simulink model "IEEE39_IBR_FrequencyControl_Primary"  (R2024a)
settings: Solver=VariableStepAuto  StartTime=0.0  StopTime=30  RelTol=1e-3
InitFcn:
  | IEEE39data_FrencyControl_primary;
values from neighbouring files (symbols this model uses):
  Fref = 60    [IEEE39data_FrencyControl_primary.m]
  IBR_data = [ ... (first row only)    [IEEE39data_FrencyControl_primary.m]
  line = [     1	2	0.0035	0.0411	0.6987	0	100	22 ... (first row only)    [IEEE39data_FrencyControl_primary.m]
  Sbase = 1e6    (= 1000000)    [IEEE39data_FrencyControl_primary.m]
  Vbase = 22e3    (= 22000)    [IEEE39data_FrencyControl_primary.m]
undefined symbols (not defined in the file or in its folder): t_start_disturbance
libraries: spsThreePhaseVIMeasurementLib x61, spsThreePhasePISectionLineLib x34, spsControlledVoltageSourceLib x33, spsabctodq0Lib x33, powerlib_extras x27, spsPLL3phLib x26, spsGroundLib x22, spsThreePhaseSeriesRLCBranchLib x22, spsThreePhaseParallelRLCLoadLib x20, slpidlib x14, spsMeanLib x11, spsdq0toabcLib x11
(part 4 of 5)

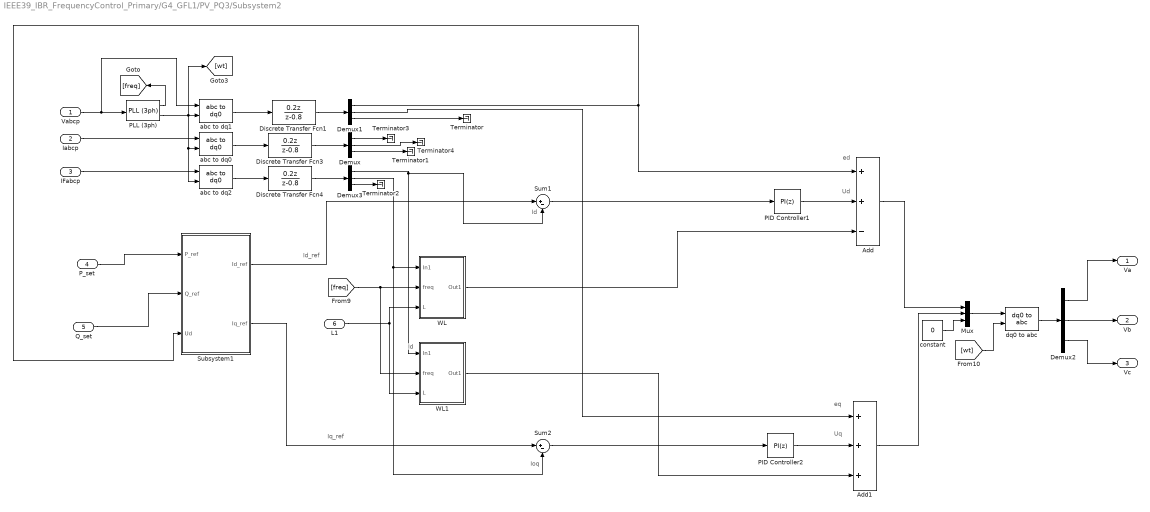
== system IEEE39_IBR_FrequencyControl_Primary/G4_GFL1/PV_PQ3/Subsystem2 ==
  note: Iq_ref
  note: Id
  note: Id_ref
  note: Ud
  note: Uq
  note: eq
  note: ed
  note: Ioq
  note: Id
  Vabcp : Inport
  Iabcp : Inport  Port=2
  IFabcp : Inport  Port=3
  P_set : Inport  Port=4
  Q_set : Inport  Port=5
  L1 : Inport  Port=6
  Add : Sum  Inputs=++-
  Add1 : Sum  Inputs=+++
  Demux{,1..3} (4 alike) : Demux  Outputs=3
  Discrete Transfer Fcn1 : DiscreteTransferFcn  Numerator=[0.2 0]  Denominator=[1 -0.8]  InitialStates=[1 1 1]  SampleTime=5e-4
  Discrete Transfer Fcn3 : DiscreteTransferFcn  Numerator=[0.2 0]  Denominator=[1 -0.8]  SampleTime=5e-4
  Discrete Transfer Fcn4 : DiscreteTransferFcn  Numerator=[0.2 0]  Denominator=[1 -0.8]  SampleTime=5e-4
  Mux : Mux  Inputs=3
  PID Controller1 : slpidlib/PID Controller  Controller=PI  Form=Parallel  TimeDomain=Discrete-time  UseExternalTs=off  SampleTime=5e-4  IntegratorMethod=Forward Euler  FilterMethod=Forward Euler  ControllerParametersSource=internal  P=50  I=400  UseKiTs=off  D=0  UseExternalDerivativeSource=off  N=100  UseFilter=on  TunerSelectOption=Transfer Function Based (PID Tuner App)  InitialConditionSource=internal  InitialConditionForIntegrator=0  InitialConditionForFilter=0  DifferentiatorICPrevScaledInput=0  ExternalReset=none  TrackingMode=off  Kt=1  LimitOutput=off  SatLimitsSource=internal  UpperSaturationLimit=inf  LowerSaturationLimit=-inf  LinearizeAsGain=on  AntiWindupMode=none  Kb=1  LimitIntegrator=off  UpperIntegratorSaturationLimit=inf  LowerIntegratorSaturationLimit=-inf  POutMin=[]  POutMax=[]  IOutMin=[]  IOutMax=[]  DOutMin=[]  DOutMax=[]  NOutMin=[]  NOutMax=[]  SumOutMin=[]  SumOutMax=[]  SaturationOutMin=[]  SaturationOutMax=[]  PParamMin=[]  PParamMax=[]  IParamMin=[]  IParamMax=[]  DParamMin=[]  DParamMax=[]  NParamMin=[]  NParamMax=[]  KbParamMin=[]  KbParamMax=[]  KtParamMin=[]  KtParamMax=[]  KbOutMin=[]  KbOutMax=[]  KtOutMin=[]  KtOutMax=[]  IntegratorOutMin=[]  IntegratorOutMax=[]  FilterOutMin=[]  FilterOutMax=[]  SumI1OutMin=[]  SumI1OutMax=[]  SumI2OutMin=[]  SumI2OutMax=[]  SumI3OutMin=[]  SumI3OutMax=[]  SumI4OutMin=[]  SumI4OutMax=[]  SumDOutMin=[]  SumDOutMax=[]  DifferentiatorOutMin=[]  DifferentiatorOutMax=[]  FilterDiffOutCoefMin=[]  FilterDiffOutCoefMax=[]  ReciprocalOutMin=[]  ReciprocalOutMax=[]  SumDenOutMin=[]  SumDenOutMax=[]  SumNumOutMin=[]  SumNumOutMax=[]  DivideOutMin=[]  DivideOutMax=[]  UdiffTsProdOutMin=[]  UdiffTsProdOutMax=[]  NTsProdOutMin=[]  NTsProdOutMax=[]  UintegralTsProdOutMin=[]  UintegralTsProdOutMax=[]  UngainTsProdOutMin=[]  UngainTsProdOutMax=[]  ClampingZeroOutDataTypeStr=Inherit: Inherit via back propagation  ClampingZeroOutMin=[]  ClampingZeroOutMax=[]  FilterDenConstantOutDataTypeStr=Inherit: Inherit via back propagation  FilterDenConstantOutMin=[]  FilterDenConstantOutMax=[]  PCopyOutDataTypeStr=Inherit: Inherit via back propagation  PCopyOutMin=[]  PCopyOutMax=[]  NCopyOutDataTypeStr=Inherit: Inherit via back propagation  NCopyOutMin=[]  NCopyOutMax=[]  IntegratorContinuousStateAttributes=''  IntegratorStateMustResolveToSignalObject=off  IntegratorRTWStateStorageClass=Auto  FilterContinuousStateAttributes=''  FilterStateMustResolveToSignalObject=off  FilterRTWStateStorageClass=Auto  ParallelPVariant=InternalParameters  IdealPVariant=Disabled  IVariant=InternalParameters  DVariant=Disabled  IntegratorVariant=Discrete  SatVariant=Disabled  AWVariant=Passthrough  PCopyVariant=Disabled  TRVariant=Disabled  FdbkBlocksVariant=Forward  IdealPFdbkVariant=Disabled  SatFdbkVariant=Disabled  DerivativeFilterVariant=Disabled  NVariant=Disabled  NCopyVariant=Disabled_SignalSpec  FilterICVariant=Disabled  IntegratorICVariant=InternalICs  ExternalResetVariant=Disabled  TRSumVariant=Passthrough  SumFdbkVariant=Disabled  SumVariant=Sum_PI  TsampFilterVariant=InternalTs  TsampNgainVariant=Passthrough  TsampIntegralVariant=Disabled_SignalSpec  ExternalSaturationOutDataTypeStr=Inherit: Same as second input  DerivativeSourceVariant=Disabled
  PID Controller2 : slpidlib/PID Controller  Controller=PI  Form=Parallel  TimeDomain=Discrete-time  UseExternalTs=off  SampleTime=5e-4  IntegratorMethod=Forward Euler  FilterMethod=Forward Euler  ControllerParametersSource=internal  P=50  I=400  UseKiTs=off  D=0  UseExternalDerivativeSource=off  N=100  UseFilter=on  TunerSelectOption=Transfer Function Based (PID Tuner App)  InitialConditionSource=internal  InitialConditionForIntegrator=0  InitialConditionForFilter=0  DifferentiatorICPrevScaledInput=0  ExternalReset=none  TrackingMode=off  Kt=1  LimitOutput=off  SatLimitsSource=internal  UpperSaturationLimit=inf  LowerSaturationLimit=-inf  LinearizeAsGain=on  AntiWindupMode=none  Kb=1  LimitIntegrator=off  UpperIntegratorSaturationLimit=inf  LowerIntegratorSaturationLimit=-inf  POutMin=[]  POutMax=[]  IOutMin=[]  IOutMax=[]  DOutMin=[]  DOutMax=[]  NOutMin=[]  NOutMax=[]  SumOutMin=[]  SumOutMax=[]  SaturationOutMin=[]  SaturationOutMax=[]  PParamMin=[]  PParamMax=[]  IParamMin=[]  IParamMax=[]  DParamMin=[]  DParamMax=[]  NParamMin=[]  NParamMax=[]  KbParamMin=[]  KbParamMax=[]  KtParamMin=[]  KtParamMax=[]  KbOutMin=[]  KbOutMax=[]  KtOutMin=[]  KtOutMax=[]  IntegratorOutMin=[]  IntegratorOutMax=[]  FilterOutMin=[]  FilterOutMax=[]  SumI1OutMin=[]  SumI1OutMax=[]  SumI2OutMin=[]  SumI2OutMax=[]  SumI3OutMin=[]  SumI3OutMax=[]  SumI4OutMin=[]  SumI4OutMax=[]  SumDOutMin=[]  SumDOutMax=[]  DifferentiatorOutMin=[]  DifferentiatorOutMax=[]  FilterDiffOutCoefMin=[]  FilterDiffOutCoefMax=[]  ReciprocalOutMin=[]  ReciprocalOutMax=[]  SumDenOutMin=[]  SumDenOutMax=[]  SumNumOutMin=[]  SumNumOutMax=[]  DivideOutMin=[]  DivideOutMax=[]  UdiffTsProdOutMin=[]  UdiffTsProdOutMax=[]  NTsProdOutMin=[]  NTsProdOutMax=[]  UintegralTsProdOutMin=[]  UintegralTsProdOutMax=[]  UngainTsProdOutMin=[]  UngainTsProdOutMax=[]  ClampingZeroOutDataTypeStr=Inherit: Inherit via back propagation  ClampingZeroOutMin=[]  ClampingZeroOutMax=[]  FilterDenConstantOutDataTypeStr=Inherit: Inherit via back propagation  FilterDenConstantOutMin=[]  FilterDenConstantOutMax=[]  PCopyOutDataTypeStr=Inherit: Inherit via back propagation  PCopyOutMin=[]  PCopyOutMax=[]  NCopyOutDataTypeStr=Inherit: Inherit via back propagation  NCopyOutMin=[]  NCopyOutMax=[]  IntegratorContinuousStateAttributes=''  IntegratorStateMustResolveToSignalObject=off  IntegratorRTWStateStorageClass=Auto  FilterContinuousStateAttributes=''  FilterStateMustResolveToSignalObject=off  FilterRTWStateStorageClass=Auto  ParallelPVariant=InternalParameters  IdealPVariant=Disabled  IVariant=InternalParameters  DVariant=Disabled  IntegratorVariant=Discrete  SatVariant=Disabled  AWVariant=Passthrough  PCopyVariant=Disabled  TRVariant=Disabled  FdbkBlocksVariant=Forward  IdealPFdbkVariant=Disabled  SatFdbkVariant=Disabled  DerivativeFilterVariant=Disabled  NVariant=Disabled  NCopyVariant=Disabled_SignalSpec  FilterICVariant=Disabled  IntegratorICVariant=InternalICs  ExternalResetVariant=Disabled  TRSumVariant=Passthrough  SumFdbkVariant=Disabled  SumVariant=Sum_PI  TsampFilterVariant=InternalTs  TsampNgainVariant=Passthrough  TsampIntegralVariant=Disabled_SignalSpec  ExternalSaturationOutDataTypeStr=Inherit: Same as second input  DerivativeSourceVariant=Disabled
  PLL (3ph) : spsPLL3phLib/PLL (3ph)  Fmin=59.5  Par_Init=[0, 60]  ParK=[180, 3200, 1]  TcD=1e-4  MaxRateChangeFreq=12  FilterCutOffFreq=25  Ts=1e-5  AGC=on
  Subsystem1 : Subsystem
  Sum1 : Sum  Inputs=|+-
  Sum2 : Sum  Inputs=|+-
  Terminator{,1..4} (5 alike) : Terminator
  WL : Subsystem
  WL1 : Subsystem
  abc to dq0 : spsabctodq0Lib/abc to dq0  Alignment=90 degrees behind phase A axis
  abc to dq1 : spsabctodq0Lib/abc to dq0  Alignment=90 degrees behind phase A axis
  abc to dq2 : spsabctodq0Lib/abc to dq0  Alignment=90 degrees behind phase A axis
  constant : Constant  Value=0
  dq0 to abc : spsdq0toabcLib/dq0 to abc  Alignment=90 degrees behind phase A axis
  Va : Outport  VectorParamsAs1DForOutWhenUnconnected=off
  Vb : Outport  Port=2  VectorParamsAs1DForOutWhenUnconnected=off
  Vc : Outport  Port=3  VectorParamsAs1DForOutWhenUnconnected=off
  wires:
  abc to dq0/1 -> Discrete Transfer Fcn3/1
  PLL (3ph)/2 -> [wt], abc to dq1/2, abc to dq2/2, abc to dq0/2
  Demux1/1 -> Add/1, Subsystem1/3(Ud)
  L1/1 -> WL/3(L), WL1/3(L)
  WL/1(Out1) -> Add/3
  [freq] -> WL1/2(freq), WL/2(freq)
  PLL (3ph)/1 -> [freq]
  Demux2/1 -> Va/1
  Add/1 -> Mux/1
  PID Controller2/1 -> Add1/2
  Demux2/2 -> Vb/1
  WL1/1(Out1) -> Add1/3
  Demux1/2 -> Add1/1
  Add1/1 -> Mux/2
  Mux/1 -> dq0 to abc/1
  Demux2/3 -> Vc/1
  dq0 to abc/1 -> Demux2/1
  Subsystem1/1(Id_ref) -> Sum1/1
  PID Controller1/1 -> Add/2
  [wt] -> dq0 to abc/2
  Subsystem1/2(Iq_ref) -> Sum2/1
  Demux1/3 -> Terminator/1
  Demux/3 -> Terminator1/1
  constant/1 -> Mux/3
  IFabcp/1 -> abc to dq2/1
  abc to dq2/1 -> Discrete Transfer Fcn4/1
  Demux3/3 -> Terminator2/1
  Demux3/2 -> Sum2/2, WL/1(In1)
  Demux3/1 -> Sum1/2, WL1/1(In1)
  Sum1/1 -> PID Controller1/1
  Sum2/1 -> PID Controller2/1
  P_set/1 -> Subsystem1/1(P_ref)
  Q_set/1 -> Subsystem1/2(Q_ref)
  Discrete Transfer Fcn3/1 -> Demux/1
  Discrete Transfer Fcn4/1 -> Demux3/1
  Demux/1 -> Terminator3/1
  Demux/2 -> Terminator4/1
  Discrete Transfer Fcn1/1 -> Demux1/1
  Iabcp/1 -> abc to dq0/1
  Vabcp/1 -> abc to dq1/1, PLL (3ph)/1
  abc to dq1/1 -> Discrete Transfer Fcn1/1

== system IEEE39_IBR_FrequencyControl_Primary/G5_GFL/PV_PQ3/Freq_Droop ==
  Pref : Inport
  Fref : Inport  Port=2
  Freq : Inport  Port=3
  D : Inport  Port=4
  Divide : Product  Inputs=*/
  Product : Product
  Product1 : Product
  S_base : Constant  Value=Sbase
  Saturation : Saturate  UpperLimit=10*Sbase  LowerLimit=0  ZeroCross=off
  Sum : Sum  Inputs=|+-
  Sum1 : Sum  Inputs=|+-
  Transfer Fcn : TransferFcn  Denominator=[0.318 1]
  Pset : Outport
  wires:
  Freq/1 -> Sum/1
  Fref/1 -> Sum/2, Divide/2
  S_base/1 -> Product/2
  D/1 -> Product1/1
  Product/1 -> Product1/2
  Pref/1 -> Sum1/1
  Product1/1 -> Sum1/2
  Saturation/1 -> Pset/1
  Sum1/1 -> Saturation/1
  Sum/1 -> Divide/1
  Transfer Fcn/1 -> Product/1
  Divide/1 -> Transfer Fcn/1

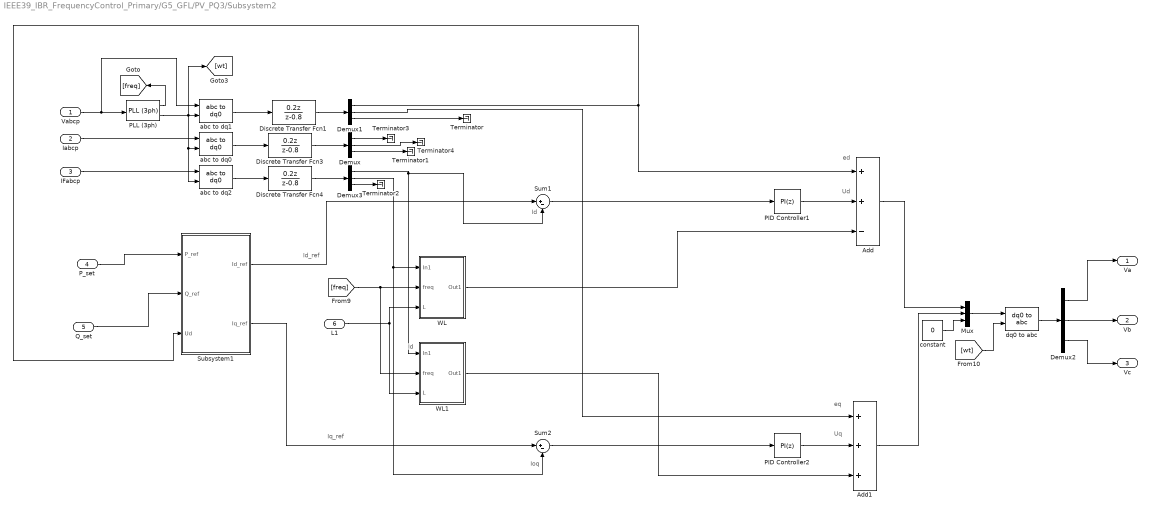
== system IEEE39_IBR_FrequencyControl_Primary/G5_GFL/PV_PQ3/Subsystem2 ==
  note: Iq_ref
  note: Id
  note: Id_ref
  note: Ud
  note: Uq
  note: eq
  note: ed
  note: Ioq
  note: Id
  Vabcp : Inport
  Iabcp : Inport  Port=2
  IFabcp : Inport  Port=3
  P_set : Inport  Port=4
  Q_set : Inport  Port=5
  L1 : Inport  Port=6
  Add : Sum  Inputs=++-
  Add1 : Sum  Inputs=+++
  Demux{,1..3} (4 alike) : Demux  Outputs=3
  Discrete Transfer Fcn1 : DiscreteTransferFcn  Numerator=[0.2 0]  Denominator=[1 -0.8]  InitialStates=[1 1 1]  SampleTime=5e-4
  Discrete Transfer Fcn3 : DiscreteTransferFcn  Numerator=[0.2 0]  Denominator=[1 -0.8]  SampleTime=5e-4
  Discrete Transfer Fcn4 : DiscreteTransferFcn  Numerator=[0.2 0]  Denominator=[1 -0.8]  SampleTime=5e-4
  Mux : Mux  Inputs=3
  PID Controller1 : slpidlib/PID Controller  Controller=PI  Form=Parallel  TimeDomain=Discrete-time  UseExternalTs=off  SampleTime=5e-4  IntegratorMethod=Forward Euler  FilterMethod=Forward Euler  ControllerParametersSource=internal  P=100  I=400  UseKiTs=off  D=0  UseExternalDerivativeSource=off  N=100  UseFilter=on  TunerSelectOption=Transfer Function Based (PID Tuner App)  InitialConditionSource=internal  InitialConditionForIntegrator=0  InitialConditionForFilter=0  DifferentiatorICPrevScaledInput=0  ExternalReset=none  TrackingMode=off  Kt=1  LimitOutput=off  SatLimitsSource=internal  UpperSaturationLimit=inf  LowerSaturationLimit=-inf  LinearizeAsGain=on  AntiWindupMode=none  Kb=1  LimitIntegrator=off  UpperIntegratorSaturationLimit=inf  LowerIntegratorSaturationLimit=-inf  POutMin=[]  POutMax=[]  IOutMin=[]  IOutMax=[]  DOutMin=[]  DOutMax=[]  NOutMin=[]  NOutMax=[]  SumOutMin=[]  SumOutMax=[]  SaturationOutMin=[]  SaturationOutMax=[]  PParamMin=[]  PParamMax=[]  IParamMin=[]  IParamMax=[]  DParamMin=[]  DParamMax=[]  NParamMin=[]  NParamMax=[]  KbParamMin=[]  KbParamMax=[]  KtParamMin=[]  KtParamMax=[]  KbOutMin=[]  KbOutMax=[]  KtOutMin=[]  KtOutMax=[]  IntegratorOutMin=[]  IntegratorOutMax=[]  FilterOutMin=[]  FilterOutMax=[]  SumI1OutMin=[]  SumI1OutMax=[]  SumI2OutMin=[]  SumI2OutMax=[]  SumI3OutMin=[]  SumI3OutMax=[]  SumI4OutMin=[]  SumI4OutMax=[]  SumDOutMin=[]  SumDOutMax=[]  DifferentiatorOutMin=[]  DifferentiatorOutMax=[]  FilterDiffOutCoefMin=[]  FilterDiffOutCoefMax=[]  ReciprocalOutMin=[]  ReciprocalOutMax=[]  SumDenOutMin=[]  SumDenOutMax=[]  SumNumOutMin=[]  SumNumOutMax=[]  DivideOutMin=[]  DivideOutMax=[]  UdiffTsProdOutMin=[]  UdiffTsProdOutMax=[]  NTsProdOutMin=[]  NTsProdOutMax=[]  UintegralTsProdOutMin=[]  UintegralTsProdOutMax=[]  UngainTsProdOutMin=[]  UngainTsProdOutMax=[]  ClampingZeroOutDataTypeStr=Inherit: Inherit via back propagation  ClampingZeroOutMin=[]  ClampingZeroOutMax=[]  FilterDenConstantOutDataTypeStr=Inherit: Inherit via back propagation  FilterDenConstantOutMin=[]  FilterDenConstantOutMax=[]  PCopyOutDataTypeStr=Inherit: Inherit via back propagation  PCopyOutMin=[]  PCopyOutMax=[]  NCopyOutDataTypeStr=Inherit: Inherit via back propagation  NCopyOutMin=[]  NCopyOutMax=[]  IntegratorContinuousStateAttributes=''  IntegratorStateMustResolveToSignalObject=off  IntegratorRTWStateStorageClass=Auto  FilterContinuousStateAttributes=''  FilterStateMustResolveToSignalObject=off  FilterRTWStateStorageClass=Auto  ParallelPVariant=InternalParameters  IdealPVariant=Disabled  IVariant=InternalParameters  DVariant=Disabled  IntegratorVariant=Discrete  SatVariant=Disabled  AWVariant=Passthrough  PCopyVariant=Disabled  TRVariant=Disabled  FdbkBlocksVariant=Forward  IdealPFdbkVariant=Disabled  SatFdbkVariant=Disabled  DerivativeFilterVariant=Disabled  NVariant=Disabled  NCopyVariant=Disabled_SignalSpec  FilterICVariant=Disabled  IntegratorICVariant=InternalICs  ExternalResetVariant=Disabled  TRSumVariant=Passthrough  SumFdbkVariant=Disabled  SumVariant=Sum_PI  TsampFilterVariant=InternalTs  TsampNgainVariant=Passthrough  TsampIntegralVariant=Disabled_SignalSpec  ExternalSaturationOutDataTypeStr=Inherit: Same as second input  DerivativeSourceVariant=Disabled
  PID Controller2 : slpidlib/PID Controller  Controller=PI  Form=Parallel  TimeDomain=Discrete-time  UseExternalTs=off  SampleTime=5e-4  IntegratorMethod=Forward Euler  FilterMethod=Forward Euler  ControllerParametersSource=internal  P=100  I=400  UseKiTs=off  D=0  UseExternalDerivativeSource=off  N=100  UseFilter=on  TunerSelectOption=Transfer Function Based (PID Tuner App)  InitialConditionSource=internal  InitialConditionForIntegrator=0  InitialConditionForFilter=0  DifferentiatorICPrevScaledInput=0  ExternalReset=none  TrackingMode=off  Kt=1  LimitOutput=off  SatLimitsSource=internal  UpperSaturationLimit=inf  LowerSaturationLimit=-inf  LinearizeAsGain=on  AntiWindupMode=none  Kb=1  LimitIntegrator=off  UpperIntegratorSaturationLimit=inf  LowerIntegratorSaturationLimit=-inf  POutMin=[]  POutMax=[]  IOutMin=[]  IOutMax=[]  DOutMin=[]  DOutMax=[]  NOutMin=[]  NOutMax=[]  SumOutMin=[]  SumOutMax=[]  SaturationOutMin=[]  SaturationOutMax=[]  PParamMin=[]  PParamMax=[]  IParamMin=[]  IParamMax=[]  DParamMin=[]  DParamMax=[]  NParamMin=[]  NParamMax=[]  KbParamMin=[]  KbParamMax=[]  KtParamMin=[]  KtParamMax=[]  KbOutMin=[]  KbOutMax=[]  KtOutMin=[]  KtOutMax=[]  IntegratorOutMin=[]  IntegratorOutMax=[]  FilterOutMin=[]  FilterOutMax=[]  SumI1OutMin=[]  SumI1OutMax=[]  SumI2OutMin=[]  SumI2OutMax=[]  SumI3OutMin=[]  SumI3OutMax=[]  SumI4OutMin=[]  SumI4OutMax=[]  SumDOutMin=[]  SumDOutMax=[]  DifferentiatorOutMin=[]  DifferentiatorOutMax=[]  FilterDiffOutCoefMin=[]  FilterDiffOutCoefMax=[]  ReciprocalOutMin=[]  ReciprocalOutMax=[]  SumDenOutMin=[]  SumDenOutMax=[]  SumNumOutMin=[]  SumNumOutMax=[]  DivideOutMin=[]  DivideOutMax=[]  UdiffTsProdOutMin=[]  UdiffTsProdOutMax=[]  NTsProdOutMin=[]  NTsProdOutMax=[]  UintegralTsProdOutMin=[]  UintegralTsProdOutMax=[]  UngainTsProdOutMin=[]  UngainTsProdOutMax=[]  ClampingZeroOutDataTypeStr=Inherit: Inherit via back propagation  ClampingZeroOutMin=[]  ClampingZeroOutMax=[]  FilterDenConstantOutDataTypeStr=Inherit: Inherit via back propagation  FilterDenConstantOutMin=[]  FilterDenConstantOutMax=[]  PCopyOutDataTypeStr=Inherit: Inherit via back propagation  PCopyOutMin=[]  PCopyOutMax=[]  NCopyOutDataTypeStr=Inherit: Inherit via back propagation  NCopyOutMin=[]  NCopyOutMax=[]  IntegratorContinuousStateAttributes=''  IntegratorStateMustResolveToSignalObject=off  IntegratorRTWStateStorageClass=Auto  FilterContinuousStateAttributes=''  FilterStateMustResolveToSignalObject=off  FilterRTWStateStorageClass=Auto  ParallelPVariant=InternalParameters  IdealPVariant=Disabled  IVariant=InternalParameters  DVariant=Disabled  IntegratorVariant=Discrete  SatVariant=Disabled  AWVariant=Passthrough  PCopyVariant=Disabled  TRVariant=Disabled  FdbkBlocksVariant=Forward  IdealPFdbkVariant=Disabled  SatFdbkVariant=Disabled  DerivativeFilterVariant=Disabled  NVariant=Disabled  NCopyVariant=Disabled_SignalSpec  FilterICVariant=Disabled  IntegratorICVariant=InternalICs  ExternalResetVariant=Disabled  TRSumVariant=Passthrough  SumFdbkVariant=Disabled  SumVariant=Sum_PI  TsampFilterVariant=InternalTs  TsampNgainVariant=Passthrough  TsampIntegralVariant=Disabled_SignalSpec  ExternalSaturationOutDataTypeStr=Inherit: Same as second input  DerivativeSourceVariant=Disabled
  PLL (3ph) : spsPLL3phLib/PLL (3ph)  Fmin=59.5  Par_Init=[0, 60]  ParK=[180, 3200, 1]  TcD=1e-4  MaxRateChangeFreq=12  FilterCutOffFreq=25  Ts=1e-5  AGC=on
  Subsystem1 : Subsystem
  Sum1 : Sum  Inputs=|+-
  Sum2 : Sum  Inputs=|+-
  Terminator{,1..4} (5 alike) : Terminator
  WL : Subsystem
  WL1 : Subsystem
  abc to dq0 : spsabctodq0Lib/abc to dq0  Alignment=90 degrees behind phase A axis
  abc to dq1 : spsabctodq0Lib/abc to dq0  Alignment=90 degrees behind phase A axis
  abc to dq2 : spsabctodq0Lib/abc to dq0  Alignment=90 degrees behind phase A axis
  constant : Constant  Value=0
  dq0 to abc : spsdq0toabcLib/dq0 to abc  Alignment=90 degrees behind phase A axis
  Va : Outport  VectorParamsAs1DForOutWhenUnconnected=off
  Vb : Outport  Port=2  VectorParamsAs1DForOutWhenUnconnected=off
  Vc : Outport  Port=3  VectorParamsAs1DForOutWhenUnconnected=off
  wires:
  abc to dq0/1 -> Discrete Transfer Fcn3/1
  PLL (3ph)/2 -> [wt], abc to dq1/2, abc to dq2/2, abc to dq0/2
  Demux1/1 -> Add/1, Subsystem1/3(Ud)
  L1/1 -> WL/3(L), WL1/3(L)
  WL/1(Out1) -> Add/3
  [freq] -> WL1/2(freq), WL/2(freq)
  PLL (3ph)/1 -> [freq]
  Demux2/1 -> Va/1
  Add/1 -> Mux/1
  PID Controller2/1 -> Add1/2
  Demux2/2 -> Vb/1
  WL1/1(Out1) -> Add1/3
  Demux1/2 -> Add1/1
  Add1/1 -> Mux/2
  Mux/1 -> dq0 to abc/1
  Demux2/3 -> Vc/1
  dq0 to abc/1 -> Demux2/1
  Subsystem1/1(Id_ref) -> Sum1/1
  PID Controller1/1 -> Add/2
  [wt] -> dq0 to abc/2
  Subsystem1/2(Iq_ref) -> Sum2/1
  Demux1/3 -> Terminator/1
  Demux/3 -> Terminator1/1
  constant/1 -> Mux/3
  IFabcp/1 -> abc to dq2/1
  abc to dq2/1 -> Discrete Transfer Fcn4/1
  Demux3/3 -> Terminator2/1
  Demux3/2 -> Sum2/2, WL/1(In1)
  Demux3/1 -> Sum1/2, WL1/1(In1)
  Sum1/1 -> PID Controller1/1
  Sum2/1 -> PID Controller2/1
  P_set/1 -> Subsystem1/1(P_ref)
  Q_set/1 -> Subsystem1/2(Q_ref)
  Discrete Transfer Fcn3/1 -> Demux/1
  Discrete Transfer Fcn4/1 -> Demux3/1
  Demux/1 -> Terminator3/1
  Demux/2 -> Terminator4/1
  Discrete Transfer Fcn1/1 -> Demux1/1
  Iabcp/1 -> abc to dq0/1
  Vabcp/1 -> abc to dq1/1, PLL (3ph)/1
  abc to dq1/1 -> Discrete Transfer Fcn1/1

== system IEEE39_IBR_FrequencyControl_Primary/G6_GFL/PV_PQ3/Freq_Droop ==
  Pref : Inport
  Fref : Inport  Port=2
  Freq : Inport  Port=3
  D : Inport  Port=4
  Divide : Product  Inputs=*/
  Product : Product
  Product1 : Product
  S_base : Constant  Value=Sbase
  Saturation : Saturate  UpperLimit=10*Sbase  LowerLimit=0  ZeroCross=off
  Sum : Sum  Inputs=|+-
  Sum1 : Sum  Inputs=|+-
  Transfer Fcn : TransferFcn  Denominator=[0.318 1]
  Pset : Outport
  wires:
  Freq/1 -> Sum/1
  Fref/1 -> Sum/2, Divide/2
  S_base/1 -> Product/2
  D/1 -> Product1/1
  Product/1 -> Product1/2
  Pref/1 -> Sum1/1
  Product1/1 -> Sum1/2
  Saturation/1 -> Pset/1
  Sum1/1 -> Saturation/1
  Sum/1 -> Divide/1
  Transfer Fcn/1 -> Product/1
  Divide/1 -> Transfer Fcn/1

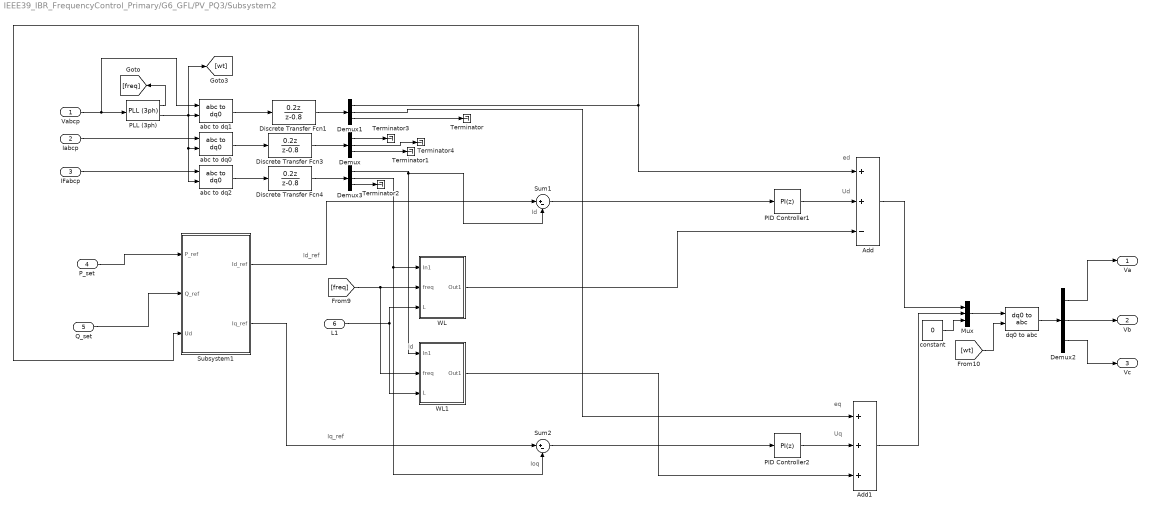
== system IEEE39_IBR_FrequencyControl_Primary/G6_GFL/PV_PQ3/Subsystem2 ==
  note: Iq_ref
  note: Id
  note: Id_ref
  note: Ud
  note: Uq
  note: eq
  note: ed
  note: Ioq
  note: Id
  Vabcp : Inport
  Iabcp : Inport  Port=2
  IFabcp : Inport  Port=3
  P_set : Inport  Port=4
  Q_set : Inport  Port=5
  L1 : Inport  Port=6
  Add : Sum  Inputs=++-
  Add1 : Sum  Inputs=+++
  Demux{,1..3} (4 alike) : Demux  Outputs=3
  Discrete Transfer Fcn1 : DiscreteTransferFcn  Numerator=[0.2 0]  Denominator=[1 -0.8]  InitialStates=[1 1 1]  SampleTime=5e-4
  Discrete Transfer Fcn3 : DiscreteTransferFcn  Numerator=[0.2 0]  Denominator=[1 -0.8]  SampleTime=5e-4
  Discrete Transfer Fcn4 : DiscreteTransferFcn  Numerator=[0.2 0]  Denominator=[1 -0.8]  SampleTime=5e-4
  Mux : Mux  Inputs=3
  PID Controller1 : slpidlib/PID Controller  Controller=PI  Form=Parallel  TimeDomain=Discrete-time  UseExternalTs=off  SampleTime=5e-4  IntegratorMethod=Forward Euler  FilterMethod=Forward Euler  ControllerParametersSource=internal  P=50  I=400  UseKiTs=off  D=0  UseExternalDerivativeSource=off  N=100  UseFilter=on  TunerSelectOption=Transfer Function Based (PID Tuner App)  InitialConditionSource=internal  InitialConditionForIntegrator=0  InitialConditionForFilter=0  DifferentiatorICPrevScaledInput=0  ExternalReset=none  TrackingMode=off  Kt=1  LimitOutput=off  SatLimitsSource=internal  UpperSaturationLimit=inf  LowerSaturationLimit=-inf  LinearizeAsGain=on  AntiWindupMode=none  Kb=1  LimitIntegrator=off  UpperIntegratorSaturationLimit=inf  LowerIntegratorSaturationLimit=-inf  POutMin=[]  POutMax=[]  IOutMin=[]  IOutMax=[]  DOutMin=[]  DOutMax=[]  NOutMin=[]  NOutMax=[]  SumOutMin=[]  SumOutMax=[]  SaturationOutMin=[]  SaturationOutMax=[]  PParamMin=[]  PParamMax=[]  IParamMin=[]  IParamMax=[]  DParamMin=[]  DParamMax=[]  NParamMin=[]  NParamMax=[]  KbParamMin=[]  KbParamMax=[]  KtParamMin=[]  KtParamMax=[]  KbOutMin=[]  KbOutMax=[]  KtOutMin=[]  KtOutMax=[]  IntegratorOutMin=[]  IntegratorOutMax=[]  FilterOutMin=[]  FilterOutMax=[]  SumI1OutMin=[]  SumI1OutMax=[]  SumI2OutMin=[]  SumI2OutMax=[]  SumI3OutMin=[]  SumI3OutMax=[]  SumI4OutMin=[]  SumI4OutMax=[]  SumDOutMin=[]  SumDOutMax=[]  DifferentiatorOutMin=[]  DifferentiatorOutMax=[]  FilterDiffOutCoefMin=[]  FilterDiffOutCoefMax=[]  ReciprocalOutMin=[]  ReciprocalOutMax=[]  SumDenOutMin=[]  SumDenOutMax=[]  SumNumOutMin=[]  SumNumOutMax=[]  DivideOutMin=[]  DivideOutMax=[]  UdiffTsProdOutMin=[]  UdiffTsProdOutMax=[]  NTsProdOutMin=[]  NTsProdOutMax=[]  UintegralTsProdOutMin=[]  UintegralTsProdOutMax=[]  UngainTsProdOutMin=[]  UngainTsProdOutMax=[]  ClampingZeroOutDataTypeStr=Inherit: Inherit via back propagation  ClampingZeroOutMin=[]  ClampingZeroOutMax=[]  FilterDenConstantOutDataTypeStr=Inherit: Inherit via back propagation  FilterDenConstantOutMin=[]  FilterDenConstantOutMax=[]  PCopyOutDataTypeStr=Inherit: Inherit via back propagation  PCopyOutMin=[]  PCopyOutMax=[]  NCopyOutDataTypeStr=Inherit: Inherit via back propagation  NCopyOutMin=[]  NCopyOutMax=[]  IntegratorContinuousStateAttributes=''  IntegratorStateMustResolveToSignalObject=off  IntegratorRTWStateStorageClass=Auto  FilterContinuousStateAttributes=''  FilterStateMustResolveToSignalObject=off  FilterRTWStateStorageClass=Auto  ParallelPVariant=InternalParameters  IdealPVariant=Disabled  IVariant=InternalParameters  DVariant=Disabled  IntegratorVariant=Discrete  SatVariant=Disabled  AWVariant=Passthrough  PCopyVariant=Disabled  TRVariant=Disabled  FdbkBlocksVariant=Forward  IdealPFdbkVariant=Disabled  SatFdbkVariant=Disabled  DerivativeFilterVariant=Disabled  NVariant=Disabled  NCopyVariant=Disabled_SignalSpec  FilterICVariant=Disabled  IntegratorICVariant=InternalICs  ExternalResetVariant=Disabled  TRSumVariant=Passthrough  SumFdbkVariant=Disabled  SumVariant=Sum_PI  TsampFilterVariant=InternalTs  TsampNgainVariant=Passthrough  TsampIntegralVariant=Disabled_SignalSpec  ExternalSaturationOutDataTypeStr=Inherit: Same as second input  DerivativeSourceVariant=Disabled
  PID Controller2 : slpidlib/PID Controller  Controller=PI  Form=Parallel  TimeDomain=Discrete-time  UseExternalTs=off  SampleTime=5e-4  IntegratorMethod=Forward Euler  FilterMethod=Forward Euler  ControllerParametersSource=internal  P=50  I=400  UseKiTs=off  D=0  UseExternalDerivativeSource=off  N=100  UseFilter=on  TunerSelectOption=Transfer Function Based (PID Tuner App)  InitialConditionSource=internal  InitialConditionForIntegrator=0  InitialConditionForFilter=0  DifferentiatorICPrevScaledInput=0  ExternalReset=none  TrackingMode=off  Kt=1  LimitOutput=off  SatLimitsSource=internal  UpperSaturationLimit=inf  LowerSaturationLimit=-inf  LinearizeAsGain=on  AntiWindupMode=none  Kb=1  LimitIntegrator=off  UpperIntegratorSaturationLimit=inf  LowerIntegratorSaturationLimit=-inf  POutMin=[]  POutMax=[]  IOutMin=[]  IOutMax=[]  DOutMin=[]  DOutMax=[]  NOutMin=[]  NOutMax=[]  SumOutMin=[]  SumOutMax=[]  SaturationOutMin=[]  SaturationOutMax=[]  PParamMin=[]  PParamMax=[]  IParamMin=[]  IParamMax=[]  DParamMin=[]  DParamMax=[]  NParamMin=[]  NParamMax=[]  KbParamMin=[]  KbParamMax=[]  KtParamMin=[]  KtParamMax=[]  KbOutMin=[]  KbOutMax=[]  KtOutMin=[]  KtOutMax=[]  IntegratorOutMin=[]  IntegratorOutMax=[]  FilterOutMin=[]  FilterOutMax=[]  SumI1OutMin=[]  SumI1OutMax=[]  SumI2OutMin=[]  SumI2OutMax=[]  SumI3OutMin=[]  SumI3OutMax=[]  SumI4OutMin=[]  SumI4OutMax=[]  SumDOutMin=[]  SumDOutMax=[]  DifferentiatorOutMin=[]  DifferentiatorOutMax=[]  FilterDiffOutCoefMin=[]  FilterDiffOutCoefMax=[]  ReciprocalOutMin=[]  ReciprocalOutMax=[]  SumDenOutMin=[]  SumDenOutMax=[]  SumNumOutMin=[]  SumNumOutMax=[]  DivideOutMin=[]  DivideOutMax=[]  UdiffTsProdOutMin=[]  UdiffTsProdOutMax=[]  NTsProdOutMin=[]  NTsProdOutMax=[]  UintegralTsProdOutMin=[]  UintegralTsProdOutMax=[]  UngainTsProdOutMin=[]  UngainTsProdOutMax=[]  ClampingZeroOutDataTypeStr=Inherit: Inherit via back propagation  ClampingZeroOutMin=[]  ClampingZeroOutMax=[]  FilterDenConstantOutDataTypeStr=Inherit: Inherit via back propagation  FilterDenConstantOutMin=[]  FilterDenConstantOutMax=[]  PCopyOutDataTypeStr=Inherit: Inherit via back propagation  PCopyOutMin=[]  PCopyOutMax=[]  NCopyOutDataTypeStr=Inherit: Inherit via back propagation  NCopyOutMin=[]  NCopyOutMax=[]  IntegratorContinuousStateAttributes=''  IntegratorStateMustResolveToSignalObject=off  IntegratorRTWStateStorageClass=Auto  FilterContinuousStateAttributes=''  FilterStateMustResolveToSignalObject=off  FilterRTWStateStorageClass=Auto  ParallelPVariant=InternalParameters  IdealPVariant=Disabled  IVariant=InternalParameters  DVariant=Disabled  IntegratorVariant=Discrete  SatVariant=Disabled  AWVariant=Passthrough  PCopyVariant=Disabled  TRVariant=Disabled  FdbkBlocksVariant=Forward  IdealPFdbkVariant=Disabled  SatFdbkVariant=Disabled  DerivativeFilterVariant=Disabled  NVariant=Disabled  NCopyVariant=Disabled_SignalSpec  FilterICVariant=Disabled  IntegratorICVariant=InternalICs  ExternalResetVariant=Disabled  TRSumVariant=Passthrough  SumFdbkVariant=Disabled  SumVariant=Sum_PI  TsampFilterVariant=InternalTs  TsampNgainVariant=Passthrough  TsampIntegralVariant=Disabled_SignalSpec  ExternalSaturationOutDataTypeStr=Inherit: Same as second input  DerivativeSourceVariant=Disabled
  PLL (3ph) : spsPLL3phLib/PLL (3ph)  Fmin=59.5  Par_Init=[0, 60]  ParK=[180, 3200, 1]  TcD=1e-4  MaxRateChangeFreq=12  FilterCutOffFreq=25  Ts=1e-5  AGC=on
  Subsystem1 : Subsystem
  Sum1 : Sum  Inputs=|+-
  Sum2 : Sum  Inputs=|+-
  Terminator{,1..4} (5 alike) : Terminator
  WL : Subsystem
  WL1 : Subsystem
  abc to dq0 : spsabctodq0Lib/abc to dq0  Alignment=90 degrees behind phase A axis
  abc to dq1 : spsabctodq0Lib/abc to dq0  Alignment=90 degrees behind phase A axis
  abc to dq2 : spsabctodq0Lib/abc to dq0  Alignment=90 degrees behind phase A axis
  constant : Constant  Value=0
  dq0 to abc : spsdq0toabcLib/dq0 to abc  Alignment=90 degrees behind phase A axis
  Va : Outport  VectorParamsAs1DForOutWhenUnconnected=off
  Vb : Outport  Port=2  VectorParamsAs1DForOutWhenUnconnected=off
  Vc : Outport  Port=3  VectorParamsAs1DForOutWhenUnconnected=off
  wires:
  abc to dq0/1 -> Discrete Transfer Fcn3/1
  PLL (3ph)/2 -> [wt], abc to dq1/2, abc to dq2/2, abc to dq0/2
  Demux1/1 -> Add/1, Subsystem1/3(Ud)
  L1/1 -> WL/3(L), WL1/3(L)
  WL/1(Out1) -> Add/3
  [freq] -> WL1/2(freq), WL/2(freq)
  PLL (3ph)/1 -> [freq]
  Demux2/1 -> Va/1
  Add/1 -> Mux/1
  PID Controller2/1 -> Add1/2
  Demux2/2 -> Vb/1
  WL1/1(Out1) -> Add1/3
  Demux1/2 -> Add1/1
  Add1/1 -> Mux/2
  Mux/1 -> dq0 to abc/1
  Demux2/3 -> Vc/1
  dq0 to abc/1 -> Demux2/1
  Subsystem1/1(Id_ref) -> Sum1/1
  PID Controller1/1 -> Add/2
  [wt] -> dq0 to abc/2
  Subsystem1/2(Iq_ref) -> Sum2/1
  Demux1/3 -> Terminator/1
  Demux/3 -> Terminator1/1
  constant/1 -> Mux/3
  IFabcp/1 -> abc to dq2/1
  abc to dq2/1 -> Discrete Transfer Fcn4/1
  Demux3/3 -> Terminator2/1
  Demux3/2 -> Sum2/2, WL/1(In1)
  Demux3/1 -> Sum1/2, WL1/1(In1)
  Sum1/1 -> PID Controller1/1
  Sum2/1 -> PID Controller2/1
  P_set/1 -> Subsystem1/1(P_ref)
  Q_set/1 -> Subsystem1/2(Q_ref)
  Discrete Transfer Fcn3/1 -> Demux/1
  Discrete Transfer Fcn4/1 -> Demux3/1
  Demux/1 -> Terminator3/1
  Demux/2 -> Terminator4/1
  Discrete Transfer Fcn1/1 -> Demux1/1
  Iabcp/1 -> abc to dq0/1
  Vabcp/1 -> abc to dq1/1, PLL (3ph)/1
  abc to dq1/1 -> Discrete Transfer Fcn1/1

== system IEEE39_IBR_FrequencyControl_Primary/GFM1/PV_PQ3/Freq_Droop ==
  Pref : Inport
  Fref : Inport  Port=2
  Pmeans : Inport  Port=3
  Add : Sum  Inputs=+-
  Add1 : Sum
  Divide : Product  Inputs=*/
  Product : Product
  S_base : Constant  Value=Sbase
  Saturation : Saturate  UpperLimit=2  LowerLimit=-2  ZeroCross=off
  Step : Step  Time=5  SampleTime=0
  Switch : Switch  Criteria=u2 > Threshold  SaturateOnIntegerOverflow=off  InputSameDT=off
  Transfer Fcn : TransferFcn  Denominator=[IBR_data(10,5) IBR_data(10,4)]
  Transfer Fcn1 : TransferFcn  Numerator=[20]  Denominator=[1 20]
  Transfer Fcn2 : TransferFcn  Denominator=[IBR_data(10,5) IBR_data(10,4)]
  fset : Outport
  wires:
  Pref/1 -> Add/1
  Transfer Fcn1/1 -> Add/2
  S_base/1 -> Divide/2
  Switch/1 -> Product/1
  Add1/1 -> fset/1
  Saturation/1 -> Add1/1
  Product/1 -> Saturation/1
  Add/1 -> Divide/1
  Pmeans/1 -> Transfer Fcn1/1
  Fref/1 -> Add1/2, Product/2
  Transfer Fcn2/1 -> Switch/1
  Transfer Fcn/1 -> Switch/3
  Step/1 -> Switch/2
  Divide/1 -> Transfer Fcn/1, Transfer Fcn2/1

== system IEEE39_IBR_FrequencyControl_Primary/GFM1/PV_PQ3/V//F ==
  vabcb : Inport
  iabcb : Inport  Port=2
  iFabcb : Inport  Port=3
  Vref_LL : Inport  Port=4
  f : Inport  Port=5
  Init_Phase_degree : Inport  Port=6
  Constant1 : Constant  Value=0
  Constant2 : Constant  Value=sqrt(2)/sqrt(3)
  Product : Product
  Subsystem : Subsystem
  UIcontrol : Subsystem
  Va : Outport
  Vb : Outport  Port=2
  Vc : Outport  Port=3
  wires:
  Constant1/1 -> UIcontrol/3(eq_ref)
  vabcb/1 -> Subsystem/1(eo)
  iFabcb/1 -> Subsystem/3(i)
  iabcb/1 -> Subsystem/2(io)
  Subsystem/1(eod) -> UIcontrol/2(ed)
  Subsystem/2(eoq) -> UIcontrol/4(eq)
  Subsystem/3(iod) -> UIcontrol/5(iod)
  Subsystem/4(ioq) -> UIcontrol/6(ioq)
  Subsystem/5(id) -> UIcontrol/7(id)
  Subsystem/6(iq) -> UIcontrol/8(iq)
  Subsystem/7(w) -> UIcontrol/9(w)
  UIcontrol/1(Va) -> Va/1
  UIcontrol/2(Vb) -> Vb/1
  UIcontrol/3(Vc) -> Vc/1
  f/1 -> Subsystem/4(f)
  Init_Phase_degree/1 -> Subsystem/5(Init_Phase_degree)
  Vref_LL/1 -> Product/1
  Product/1 -> UIcontrol/1(ed_ref)
  Constant2/1 -> Product/2
  Subsystem/8("wt ") -> UIcontrol/10("wt ")

== system IEEE39_IBR_FrequencyControl_Primary/GFM2/PV_PQ3/Freq_Droop ==
  Pref : Inport
  Fref : Inport  Port=2
  Pmeans : Inport  Port=3
  Add : Sum  Inputs=+-
  Add1 : Sum
  Divide : Product  Inputs=*/
  Product : Product
  S_base : Constant  Value=Sbase
  Saturation : Saturate  UpperLimit=2  LowerLimit=-2  ZeroCross=off
  Step : Step  Time=5  SampleTime=0
  Switch : Switch  Criteria=u2 > Threshold  SaturateOnIntegerOverflow=off  InputSameDT=off
  Transfer Fcn : TransferFcn  Denominator=[IBR_data(9,5) IBR_data(9,4)]
  Transfer Fcn1 : TransferFcn  Numerator=[20]  Denominator=[1 20]
  Transfer Fcn2 : TransferFcn  Denominator=[IBR_data(9,5) IBR_data(9,4)]
  fset : Outport
  wires:
  Pref/1 -> Add/1
  Transfer Fcn1/1 -> Add/2
  S_base/1 -> Divide/2
  Switch/1 -> Product/1
  Add1/1 -> fset/1
  Saturation/1 -> Add1/1
  Product/1 -> Saturation/1
  Add/1 -> Divide/1
  Pmeans/1 -> Transfer Fcn1/1
  Fref/1 -> Add1/2, Product/2
  Transfer Fcn2/1 -> Switch/1
  Transfer Fcn/1 -> Switch/3
  Step/1 -> Switch/2
  Divide/1 -> Transfer Fcn/1, Transfer Fcn2/1

== system IEEE39_IBR_FrequencyControl_Primary/GFM2/PV_PQ3/V//F ==
  vabcb : Inport
  iabcb : Inport  Port=2
  iFabcb : Inport  Port=3
  Vref_LL : Inport  Port=4
  f : Inport  Port=5
  Init_Phase_degree : Inport  Port=6
  Constant : Constant  Value=2*pi
  Constant1 : Constant  Value=0
  Constant2 : Constant  Value=sqrt(2)/sqrt(3)
  Divide : Product  Inputs=*/
  Product : Product
  Scope1 : Scope
  Subsystem : Subsystem
  UIcontrol : Subsystem
  Va : Outport
  Vb : Outport  Port=2
  Vc : Outport  Port=3
  wires:
  Constant1/1 -> UIcontrol/3(eq_ref)
  vabcb/1 -> Subsystem/1(eo)
  iFabcb/1 -> Subsystem/3(i)
  iabcb/1 -> Subsystem/2(io)
  Subsystem/1(eod) -> UIcontrol/2(ed)
  Subsystem/2(eoq) -> UIcontrol/4(eq)
  Subsystem/3(iod) -> UIcontrol/5(iod)
  Subsystem/4(ioq) -> UIcontrol/6(ioq)
  Subsystem/5(id) -> UIcontrol/7(id)
  Subsystem/6(iq) -> UIcontrol/8(iq)
  Subsystem/7(w) -> Divide/1, UIcontrol/9(w)
  UIcontrol/1(Va) -> Va/1
  UIcontrol/2(Vb) -> Vb/1
  UIcontrol/3(Vc) -> Vc/1
  f/1 -> Subsystem/4(f)
  Init_Phase_degree/1 -> Subsystem/5(Init_Phase_degree)
  Vref_LL/1 -> Product/1
  Product/1 -> UIcontrol/1(ed_ref)
  Constant2/1 -> Product/2
  Subsystem/8("wt ") -> UIcontrol/10("wt ")
  Constant/1 -> Divide/2
  Divide/1 -> Scope1/1

== system IEEE39_IBR_FrequencyControl_Primary/GFM3/PV_PQ3/Freq_Droop ==
  Pref : Inport
  Fref : Inport  Port=2
  Pmeans : Inport  Port=3
  Add : Sum  Inputs=+-
  Add1 : Sum
  Divide : Product  Inputs=*/
  Product : Product
  S_base : Constant  Value=Sbase
  Saturation : Saturate  UpperLimit=2  LowerLimit=-2  ZeroCross=off
  Step : Step  Time=5  SampleTime=0
  Switch : Switch  Criteria=u2 > Threshold  SaturateOnIntegerOverflow=off  InputSameDT=off
  Transfer Fcn : TransferFcn  Denominator=[IBR_data(8,5) IBR_data(8,4)]
  Transfer Fcn1 : TransferFcn  Numerator=[20]  Denominator=[1 20]
  Transfer Fcn2 : TransferFcn  Denominator=[IBR_data(8,5) IBR_data(8,4)]
  fset : Outport
  wires:
  Pref/1 -> Add/1
  Transfer Fcn1/1 -> Add/2
  S_base/1 -> Divide/2
  Switch/1 -> Product/1
  Add1/1 -> fset/1
  Saturation/1 -> Add1/1
  Product/1 -> Saturation/1
  Add/1 -> Divide/1
  Pmeans/1 -> Transfer Fcn1/1
  Fref/1 -> Add1/2, Product/2
  Transfer Fcn2/1 -> Switch/1
  Transfer Fcn/1 -> Switch/3
  Step/1 -> Switch/2
  Divide/1 -> Transfer Fcn/1, Transfer Fcn2/1

== system IEEE39_IBR_FrequencyControl_Primary/GFM3/PV_PQ3/V//F ==
  vabcb : Inport
  iabcb : Inport  Port=2
  iFabcb : Inport  Port=3
  Vref_LL : Inport  Port=4
  f : Inport  Port=5
  Init_Phase_degree : Inport  Port=6
  Constant : Constant  Value=2*pi
  Constant1 : Constant  Value=0
  Constant2 : Constant  Value=sqrt(2)/sqrt(3)
  Divide : Product  Inputs=*/
  Product : Product
  Scope1 : Scope
  Subsystem : Subsystem
  UIcontrol : Subsystem
  Va : Outport
  Vb : Outport  Port=2
  Vc : Outport  Port=3
  wires:
  Constant1/1 -> UIcontrol/3(eq_ref)
  vabcb/1 -> Subsystem/1(eo)
  iFabcb/1 -> Subsystem/3(i)
  iabcb/1 -> Subsystem/2(io)
  Subsystem/1(eod) -> UIcontrol/2(ed)
  Subsystem/2(eoq) -> UIcontrol/4(eq)
  Subsystem/3(iod) -> UIcontrol/5(iod)
  Subsystem/4(ioq) -> UIcontrol/6(ioq)
  Subsystem/5(id) -> UIcontrol/7(id)
  Subsystem/6(iq) -> UIcontrol/8(iq)
  Subsystem/7(w) -> Divide/1, UIcontrol/9(w)
  UIcontrol/1(Va) -> Va/1
  UIcontrol/2(Vb) -> Vb/1
  UIcontrol/3(Vc) -> Vc/1
  f/1 -> Subsystem/4(f)
  Init_Phase_degree/1 -> Subsystem/5(Init_Phase_degree)
  Vref_LL/1 -> Product/1
  Product/1 -> UIcontrol/1(ed_ref)
  Constant2/1 -> Product/2
  Subsystem/8("wt ") -> UIcontrol/10("wt ")
  Constant/1 -> Divide/2
  Divide/1 -> Scope1/1

== system IEEE39_IBR_FrequencyControl_Primary/GFM4/PV_PQ3/Freq_Droop ==
  Pref : Inport
  Fref : Inport  Port=2
  Pmeans : Inport  Port=3
  Add : Sum  Inputs=+-
  Add1 : Sum
  Divide : Product  Inputs=*/
  Product : Product
  S_base : Constant  Value=Sbase
  Saturation : Saturate  UpperLimit=2  LowerLimit=-2  ZeroCross=off
  Step : Step  Time=5  SampleTime=0
  Switch : Switch  Criteria=u2 > Threshold  SaturateOnIntegerOverflow=off  InputSameDT=off
  Transfer Fcn : TransferFcn  Denominator=[IBR_data(7,5) IBR_data(7,4)]
  Transfer Fcn1 : TransferFcn  Numerator=[20]  Denominator=[1 20]
  Transfer Fcn2 : TransferFcn  Denominator=[IBR_data(7,5) IBR_data(7,4)]
  fset : Outport
  wires:
  Pref/1 -> Add/1
  Transfer Fcn1/1 -> Add/2
  S_base/1 -> Divide/2
  Switch/1 -> Product/1
  Add1/1 -> fset/1
  Saturation/1 -> Add1/1
  Product/1 -> Saturation/1
  Add/1 -> Divide/1
  Pmeans/1 -> Transfer Fcn1/1
  Fref/1 -> Add1/2, Product/2
  Transfer Fcn2/1 -> Switch/1
  Transfer Fcn/1 -> Switch/3
  Step/1 -> Switch/2
  Divide/1 -> Transfer Fcn/1, Transfer Fcn2/1

== system IEEE39_IBR_FrequencyControl_Primary/GFM4/PV_PQ3/V//F ==
  vabcb : Inport
  iabcb : Inport  Port=2
  iFabcb : Inport  Port=3
  Vref_LL : Inport  Port=4
  f : Inport  Port=5
  Init_Phase_degree : Inport  Port=6
  Constant : Constant  Value=2*pi
  Constant1 : Constant  Value=0
  Constant2 : Constant  Value=sqrt(2)/sqrt(3)
  Divide : Product  Inputs=*/
  Product : Product
  Scope1 : Scope
  Subsystem : Subsystem
  UIcontrol : Subsystem
  Va : Outport
  Vb : Outport  Port=2
  Vc : Outport  Port=3
  wires:
  Constant1/1 -> UIcontrol/3(eq_ref)
  vabcb/1 -> Subsystem/1(eo)
  iFabcb/1 -> Subsystem/3(i)
  iabcb/1 -> Subsystem/2(io)
  Subsystem/1(eod) -> UIcontrol/2(ed)
  Subsystem/2(eoq) -> UIcontrol/4(eq)
  Subsystem/3(iod) -> UIcontrol/5(iod)
  Subsystem/4(ioq) -> UIcontrol/6(ioq)
  Subsystem/5(id) -> UIcontrol/7(id)
  Subsystem/6(iq) -> UIcontrol/8(iq)
  Subsystem/7(w) -> Divide/1, UIcontrol/9(w)
  UIcontrol/1(Va) -> Va/1
  UIcontrol/2(Vb) -> Vb/1
  UIcontrol/3(Vc) -> Vc/1
  f/1 -> Subsystem/4(f)
  Init_Phase_degree/1 -> Subsystem/5(Init_Phase_degree)
  Vref_LL/1 -> Product/1
  Product/1 -> UIcontrol/1(ed_ref)
  Constant2/1 -> Product/2
  Subsystem/8("wt ") -> UIcontrol/10("wt ")
  Constant/1 -> Divide/2
  Divide/1 -> Scope1/1

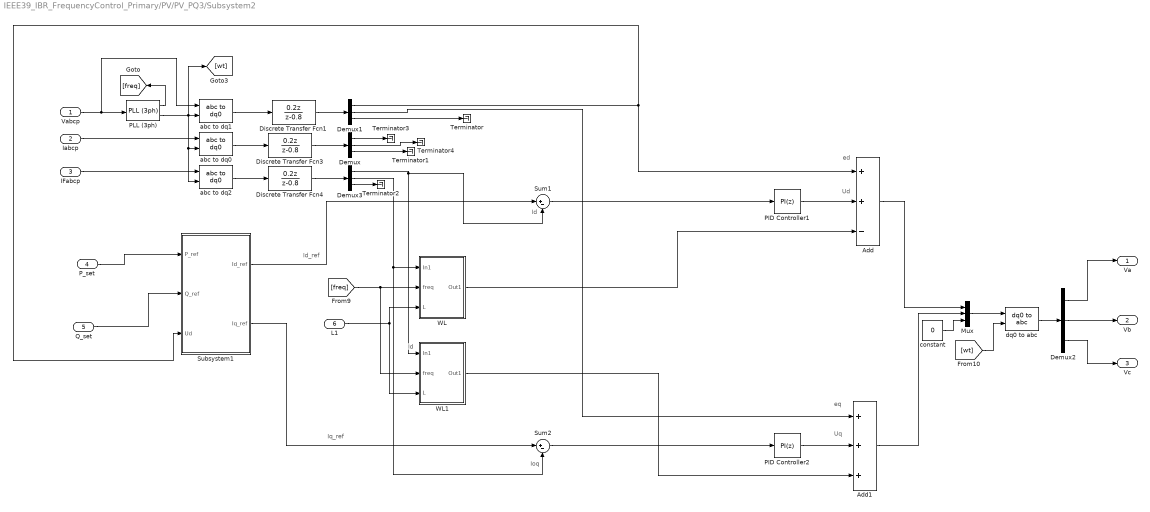
== system IEEE39_IBR_FrequencyControl_Primary/PV/PV_PQ3/Subsystem2 ==
  note: Iq_ref
  note: Id
  note: Id_ref
  note: Ud
  note: Uq
  note: eq
  note: ed
  note: Ioq
  note: Id
  Vabcp : Inport
  Iabcp : Inport  Port=2
  IFabcp : Inport  Port=3
  P_set : Inport  Port=4
  Q_set : Inport  Port=5
  L1 : Inport  Port=6
  Add : Sum  Inputs=++-
  Add1 : Sum  Inputs=+++
  Demux{,1..3} (4 alike) : Demux  Outputs=3
  Discrete Transfer Fcn1 : DiscreteTransferFcn  Numerator=[0.2 0]  Denominator=[1 -0.8]  InitialStates=[1 1 1]  SampleTime=5e-4
  Discrete Transfer Fcn3 : DiscreteTransferFcn  Numerator=[0.2 0]  Denominator=[1 -0.8]  SampleTime=5e-4
  Discrete Transfer Fcn4 : DiscreteTransferFcn  Numerator=[0.2 0]  Denominator=[1 -0.8]  SampleTime=5e-4
  Mux : Mux  Inputs=3
  PID Controller1 : slpidlib/PID Controller  Controller=PI  Form=Parallel  TimeDomain=Discrete-time  UseExternalTs=off  SampleTime=5e-4  IntegratorMethod=Forward Euler  FilterMethod=Forward Euler  ControllerParametersSource=internal  P=100  I=400  UseKiTs=off  D=0  UseExternalDerivativeSource=off  N=100  UseFilter=on  TunerSelectOption=Transfer Function Based (PID Tuner App)  InitialConditionSource=internal  InitialConditionForIntegrator=0  InitialConditionForFilter=0  DifferentiatorICPrevScaledInput=0  ExternalReset=none  TrackingMode=off  Kt=1  LimitOutput=off  SatLimitsSource=internal  UpperSaturationLimit=inf  LowerSaturationLimit=-inf  LinearizeAsGain=on  AntiWindupMode=none  Kb=1  LimitIntegrator=off  UpperIntegratorSaturationLimit=inf  LowerIntegratorSaturationLimit=-inf  POutMin=[]  POutMax=[]  IOutMin=[]  IOutMax=[]  DOutMin=[]  DOutMax=[]  NOutMin=[]  NOutMax=[]  SumOutMin=[]  SumOutMax=[]  SaturationOutMin=[]  SaturationOutMax=[]  PParamMin=[]  PParamMax=[]  IParamMin=[]  IParamMax=[]  DParamMin=[]  DParamMax=[]  NParamMin=[]  NParamMax=[]  KbParamMin=[]  KbParamMax=[]  KtParamMin=[]  KtParamMax=[]  KbOutMin=[]  KbOutMax=[]  KtOutMin=[]  KtOutMax=[]  IntegratorOutMin=[]  IntegratorOutMax=[]  FilterOutMin=[]  FilterOutMax=[]  SumI1OutMin=[]  SumI1OutMax=[]  SumI2OutMin=[]  SumI2OutMax=[]  SumI3OutMin=[]  SumI3OutMax=[]  SumI4OutMin=[]  SumI4OutMax=[]  SumDOutMin=[]  SumDOutMax=[]  DifferentiatorOutMin=[]  DifferentiatorOutMax=[]  FilterDiffOutCoefMin=[]  FilterDiffOutCoefMax=[]  ReciprocalOutMin=[]  ReciprocalOutMax=[]  SumDenOutMin=[]  SumDenOutMax=[]  SumNumOutMin=[]  SumNumOutMax=[]  DivideOutMin=[]  DivideOutMax=[]  UdiffTsProdOutMin=[]  UdiffTsProdOutMax=[]  NTsProdOutMin=[]  NTsProdOutMax=[]  UintegralTsProdOutMin=[]  UintegralTsProdOutMax=[]  UngainTsProdOutMin=[]  UngainTsProdOutMax=[]  ClampingZeroOutDataTypeStr=Inherit: Inherit via back propagation  ClampingZeroOutMin=[]  ClampingZeroOutMax=[]  FilterDenConstantOutDataTypeStr=Inherit: Inherit via back propagation  FilterDenConstantOutMin=[]  FilterDenConstantOutMax=[]  PCopyOutDataTypeStr=Inherit: Inherit via back propagation  PCopyOutMin=[]  PCopyOutMax=[]  NCopyOutDataTypeStr=Inherit: Inherit via back propagation  NCopyOutMin=[]  NCopyOutMax=[]  IntegratorContinuousStateAttributes=''  IntegratorStateMustResolveToSignalObject=off  IntegratorRTWStateStorageClass=Auto  FilterContinuousStateAttributes=''  FilterStateMustResolveToSignalObject=off  FilterRTWStateStorageClass=Auto  ParallelPVariant=InternalParameters  IdealPVariant=Disabled  IVariant=InternalParameters  DVariant=Disabled  IntegratorVariant=Discrete  SatVariant=Disabled  AWVariant=Passthrough  PCopyVariant=Disabled  TRVariant=Disabled  FdbkBlocksVariant=Forward  IdealPFdbkVariant=Disabled  SatFdbkVariant=Disabled  DerivativeFilterVariant=Disabled  NVariant=Disabled  NCopyVariant=Disabled_SignalSpec  FilterICVariant=Disabled  IntegratorICVariant=InternalICs  ExternalResetVariant=Disabled  TRSumVariant=Passthrough  SumFdbkVariant=Disabled  SumVariant=Sum_PI  TsampFilterVariant=InternalTs  TsampNgainVariant=Passthrough  TsampIntegralVariant=Disabled_SignalSpec  ExternalSaturationOutDataTypeStr=Inherit: Same as second input  DerivativeSourceVariant=Disabled
  PID Controller2 : slpidlib/PID Controller  Controller=PI  Form=Parallel  TimeDomain=Discrete-time  UseExternalTs=off  SampleTime=5e-4  IntegratorMethod=Forward Euler  FilterMethod=Forward Euler  ControllerParametersSource=internal  P=100  I=400  UseKiTs=off  D=0  UseExternalDerivativeSource=off  N=100  UseFilter=on  TunerSelectOption=Transfer Function Based (PID Tuner App)  InitialConditionSource=internal  InitialConditionForIntegrator=0  InitialConditionForFilter=0  DifferentiatorICPrevScaledInput=0  ExternalReset=none  TrackingMode=off  Kt=1  LimitOutput=off  SatLimitsSource=internal  UpperSaturationLimit=inf  LowerSaturationLimit=-inf  LinearizeAsGain=on  AntiWindupMode=none  Kb=1  LimitIntegrator=off  UpperIntegratorSaturationLimit=inf  LowerIntegratorSaturationLimit=-inf  POutMin=[]  POutMax=[]  IOutMin=[]  IOutMax=[]  DOutMin=[]  DOutMax=[]  NOutMin=[]  NOutMax=[]  SumOutMin=[]  SumOutMax=[]  SaturationOutMin=[]  SaturationOutMax=[]  PParamMin=[]  PParamMax=[]  IParamMin=[]  IParamMax=[]  DParamMin=[]  DParamMax=[]  NParamMin=[]  NParamMax=[]  KbParamMin=[]  KbParamMax=[]  KtParamMin=[]  KtParamMax=[]  KbOutMin=[]  KbOutMax=[]  KtOutMin=[]  KtOutMax=[]  IntegratorOutMin=[]  IntegratorOutMax=[]  FilterOutMin=[]  FilterOutMax=[]  SumI1OutMin=[]  SumI1OutMax=[]  SumI2OutMin=[]  SumI2OutMax=[]  SumI3OutMin=[]  SumI3OutMax=[]  SumI4OutMin=[]  SumI4OutMax=[]  SumDOutMin=[]  SumDOutMax=[]  DifferentiatorOutMin=[]  DifferentiatorOutMax=[]  FilterDiffOutCoefMin=[]  FilterDiffOutCoefMax=[]  ReciprocalOutMin=[]  ReciprocalOutMax=[]  SumDenOutMin=[]  SumDenOutMax=[]  SumNumOutMin=[]  SumNumOutMax=[]  DivideOutMin=[]  DivideOutMax=[]  UdiffTsProdOutMin=[]  UdiffTsProdOutMax=[]  NTsProdOutMin=[]  NTsProdOutMax=[]  UintegralTsProdOutMin=[]  UintegralTsProdOutMax=[]  UngainTsProdOutMin=[]  UngainTsProdOutMax=[]  ClampingZeroOutDataTypeStr=Inherit: Inherit via back propagation  ClampingZeroOutMin=[]  ClampingZeroOutMax=[]  FilterDenConstantOutDataTypeStr=Inherit: Inherit via back propagation  FilterDenConstantOutMin=[]  FilterDenConstantOutMax=[]  PCopyOutDataTypeStr=Inherit: Inherit via back propagation  PCopyOutMin=[]  PCopyOutMax=[]  NCopyOutDataTypeStr=Inherit: Inherit via back propagation  NCopyOutMin=[]  NCopyOutMax=[]  IntegratorContinuousStateAttributes=''  IntegratorStateMustResolveToSignalObject=off  IntegratorRTWStateStorageClass=Auto  FilterContinuousStateAttributes=''  FilterStateMustResolveToSignalObject=off  FilterRTWStateStorageClass=Auto  ParallelPVariant=InternalParameters  IdealPVariant=Disabled  IVariant=InternalParameters  DVariant=Disabled  IntegratorVariant=Discrete  SatVariant=Disabled  AWVariant=Passthrough  PCopyVariant=Disabled  TRVariant=Disabled  FdbkBlocksVariant=Forward  IdealPFdbkVariant=Disabled  SatFdbkVariant=Disabled  DerivativeFilterVariant=Disabled  NVariant=Disabled  NCopyVariant=Disabled_SignalSpec  FilterICVariant=Disabled  IntegratorICVariant=InternalICs  ExternalResetVariant=Disabled  TRSumVariant=Passthrough  SumFdbkVariant=Disabled  SumVariant=Sum_PI  TsampFilterVariant=InternalTs  TsampNgainVariant=Passthrough  TsampIntegralVariant=Disabled_SignalSpec  ExternalSaturationOutDataTypeStr=Inherit: Same as second input  DerivativeSourceVariant=Disabled
  PLL (3ph) : spsPLL3phLib/PLL (3ph)  Fmin=59.5  Par_Init=[0, 60]  ParK=[180, 3200, 1]  TcD=1e-4  MaxRateChangeFreq=12  FilterCutOffFreq=25  Ts=1e-5  AGC=on
  Subsystem1 : Subsystem
  Sum1 : Sum  Inputs=|+-
  Sum2 : Sum  Inputs=|+-
  Terminator{,1..4} (5 alike) : Terminator
  WL : Subsystem
  WL1 : Subsystem
  abc to dq0 : spsabctodq0Lib/abc to dq0  Alignment=90 degrees behind phase A axis
  abc to dq1 : spsabctodq0Lib/abc to dq0  Alignment=90 degrees behind phase A axis
  abc to dq2 : spsabctodq0Lib/abc to dq0  Alignment=90 degrees behind phase A axis
  constant : Constant  Value=0
  dq0 to abc : spsdq0toabcLib/dq0 to abc  Alignment=90 degrees behind phase A axis
  Va : Outport  VectorParamsAs1DForOutWhenUnconnected=off
  Vb : Outport  Port=2  VectorParamsAs1DForOutWhenUnconnected=off
  Vc : Outport  Port=3  VectorParamsAs1DForOutWhenUnconnected=off
  wires:
  abc to dq0/1 -> Discrete Transfer Fcn3/1
  PLL (3ph)/2 -> [wt], abc to dq1/2, abc to dq2/2, abc to dq0/2
  Demux1/1 -> Add/1, Subsystem1/3(Ud)
  L1/1 -> WL/3(L), WL1/3(L)
  WL/1(Out1) -> Add/3
  [freq] -> WL1/2(freq), WL/2(freq)
  PLL (3ph)/1 -> [freq]
  Demux2/1 -> Va/1
  Add/1 -> Mux/1
  PID Controller2/1 -> Add1/2
  Demux2/2 -> Vb/1
  WL1/1(Out1) -> Add1/3
  Demux1/2 -> Add1/1
  Add1/1 -> Mux/2
  Mux/1 -> dq0 to abc/1
  Demux2/3 -> Vc/1
  dq0 to abc/1 -> Demux2/1
  Subsystem1/1(Id_ref) -> Sum1/1
  PID Controller1/1 -> Add/2
  [wt] -> dq0 to abc/2
  Subsystem1/2(Iq_ref) -> Sum2/1
  Demux1/3 -> Terminator/1
  Demux/3 -> Terminator1/1
  constant/1 -> Mux/3
  IFabcp/1 -> abc to dq2/1
  abc to dq2/1 -> Discrete Transfer Fcn4/1
  Demux3/3 -> Terminator2/1
  Demux3/2 -> Sum2/2, WL/1(In1)
  Demux3/1 -> Sum1/2, WL1/1(In1)
  Sum1/1 -> PID Controller1/1
  Sum2/1 -> PID Controller2/1
  P_set/1 -> Subsystem1/1(P_ref)
  Q_set/1 -> Subsystem1/2(Q_ref)
  Discrete Transfer Fcn3/1 -> Demux/1
  Discrete Transfer Fcn4/1 -> Demux3/1
  Demux/1 -> Terminator3/1
  Demux/2 -> Terminator4/1
  Discrete Transfer Fcn1/1 -> Demux1/1
  Iabcp/1 -> abc to dq0/1
  Vabcp/1 -> abc to dq1/1, PLL (3ph)/1
  abc to dq1/1 -> Discrete Transfer Fcn1/1

== system IEEE39_IBR_FrequencyControl_Primary/G1_GFL/PV_PQ3/Subsystem2/Subsystem1 ==
  P_ref : Inport
  Q_ref : Inport  Port=2
  Ud : Inport  Port=3
  Divide5 : Product  Inputs=*/
  Divide6 : Product  Inputs=*/
  Gain1 : Gain  Gain=-2/3
  Gain2 : Gain  Gain=2/3
  Id_ref : Outport  VectorParamsAs1DForOutWhenUnconnected=off
  Iq_ref : Outport  Port=2  VectorParamsAs1DForOutWhenUnconnected=off
  wires:
  Q_ref/1 -> Divide6/1
  Divide6/1 -> Gain1/1
  P_ref/1 -> Divide5/1
  Gain1/1 -> Iq_ref/1
  Divide5/1 -> Gain2/1
  Gain2/1 -> Id_ref/1
  Ud/1 -> Divide6/2, Divide5/2
